simulink model "Kalman_kaskada"  (Simulink 7.8)
settings: Solver=ode45  StartTime=0.0  StopTime=100  RelTol=1e-3
values from neighbouring files (symbols this model uses):
  A = [-1/8 1/8 0 0; 0 -1/10 1/10 0;0 0 -1/1.2 1/1.2; 0 0 0 -1/0.8]    [Parametri.m]
  A1 = [-1/8 1/8 0 0; 0 -1/10 1/10 0;0 0 -1/1.2 1/1.2; 0 0 0 -1/0.8]    [Parametri.m]
  B = [0; 0; 0; 1/0.8]    [Parametri.m]
  B1 = [0; 0; 0; 1/0.8]    [Parametri.m]
  C = [1 0 0 0]    [Parametri.m]
  C1 = [1 0 0 0]    [Parametri.m]
  D = 0    [Parametri.m]
  P1 = 0    [Parametri.m]
  Q = 1*eye(4,4)    [Parametri.m]
  Q1 = 1*eye(4,4)    [Parametri.m]
  R = 1    [Parametri.m]
  R1 = 1    [Parametri.m]
  x0 = [0; 0; 0 ;0]    [Parametri.m]
  x10 = [0; 0; 0 ;0]    [Parametri.m]
undefined symbols (not defined in the file or in its folder): D1
libraries: simulink x4
settings Model: Creator=fo1521  LastModifiedBy=AA
settings OptimizationCC: InitFltsAndDblsToZero=on
settings DebuggingCC: SaveWithParameterizedLinksMsg=none  SolverPrmCheckMsg=none  MultiTaskCondExecSysMsg=none  FcnCallInpInsideContextMsg=Use local settings  StrictBusMsg=None
settings RTWCC: IncludeERTFirstTime=on

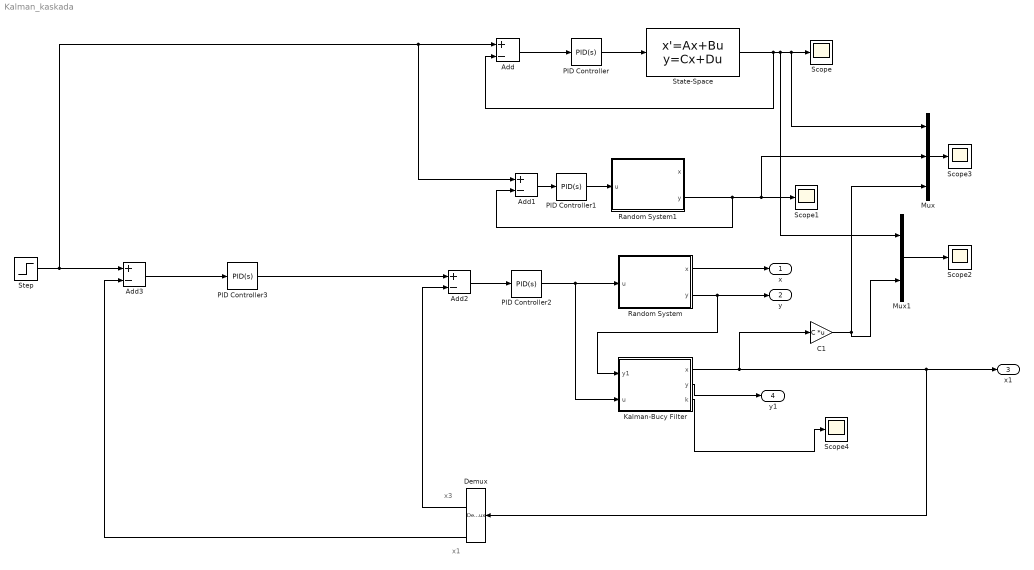
== system Kalman_kaskada ==
  note: x1
  note: x3
  Add{,1..3} (4 alike) : Sum  Inputs=+-
  C1 : Gain  Gain=C  Multiplication=Matrix(K*u)
  Demux : Demux
  Kalman-Bucy Filter : Subsystem  mask{x0=x10, P0=P1, A=A1, B=B1, C=C1, D=D1, Q=Q1, R=R1}
      mask Display:
      | port_label('input',1,'y')
      | port_label('input',2,'u')
      | port_label('output',1,'x')
      | port_label('output',2,'y')
      | disp(sprintf('Kalman-Bucy\n Filter'))
  Mux : Mux  Inputs=3
  Mux1 : Mux  Inputs=2
  PID Controller : simulink/Continuous/PID Controller  Controller=PID  TimeDomain=Continuous-time  SampleTime=1  IntegratorMethod=Forward Euler  FilterMethod=Forward Euler  Form=Parallel  P=2.29954504255598  I=0.157366537101779  D=7.23056950436541  N=1.36221313927971  InitialConditionSource=internal  InitialConditionForIntegrator=0  InitialConditionForFilter=0  ExternalReset=none  LimitOutput=off  UpperSaturationLimit=inf  LowerSaturationLimit=-inf  LinearizeAsGain=off  AntiWindupMode=none  Kb=1  TrackingMode=off  Kt=1  PParamMin=[]  PParamMax=[]  IParamMin=[]  IParamMax=[]  DParamMin=[]  DParamMax=[]  NParamMin=[]  NParamMax=[]  KbParamMin=[]  KbParamMax=[]  KtParamMin=[]  KtParamMax=[]  POutMin=[]  POutMax=[]  IOutMin=[]  IOutMax=[]  DOutMin=[]  DOutMax=[]  NOutMin=[]  NOutMax=[]  KbOutMin=[]  KbOutMax=[]  KtOutMin=[]  KtOutMax=[]  IntegratorOutMin=[]  IntegratorOutMax=[]  FilterOutMin=[]  FilterOutMax=[]  SumOutMin=[]  SumOutMax=[]  SumI1OutMin=[]  SumI1OutMax=[]  SumI2OutMin=[]  SumI2OutMax=[]  SumI3OutMin=[]  SumI3OutMax=[]  SumDOutMin=[]  SumDOutMax=[]  SaturationOutMin=[]  SaturationOutMax=[]  IntegratorContinuousStateAttributes=''  IntegratorStateMustResolveToSignalObject=off  IntegratorRTWStateStorageClass=Auto  FilterContinuousStateAttributes=''  FilterStateMustResolveToSignalObject=off  FilterRTWStateStorageClass=Auto
  PID Controller1 : simulink/Continuous/PID Controller  Controller=PID  TimeDomain=Continuous-time  SampleTime=1  IntegratorMethod=Forward Euler  FilterMethod=Forward Euler  Form=Parallel  P=1  I=1  D=1  N=100  InitialConditionSource=internal  InitialConditionForIntegrator=0  InitialConditionForFilter=0  ExternalReset=none  LimitOutput=off  UpperSaturationLimit=inf  LowerSaturationLimit=-inf  LinearizeAsGain=off  AntiWindupMode=none  Kb=1  TrackingMode=off  Kt=1  PParamMin=[]  PParamMax=[]  IParamMin=[]  IParamMax=[]  DParamMin=[]  DParamMax=[]  NParamMin=[]  NParamMax=[]  KbParamMin=[]  KbParamMax=[]  KtParamMin=[]  KtParamMax=[]  POutMin=[]  POutMax=[]  IOutMin=[]  IOutMax=[]  DOutMin=[]  DOutMax=[]  NOutMin=[]  NOutMax=[]  KbOutMin=[]  KbOutMax=[]  KtOutMin=[]  KtOutMax=[]  IntegratorOutMin=[]  IntegratorOutMax=[]  FilterOutMin=[]  FilterOutMax=[]  SumOutMin=[]  SumOutMax=[]  SumI1OutMin=[]  SumI1OutMax=[]  SumI2OutMin=[]  SumI2OutMax=[]  SumI3OutMin=[]  SumI3OutMax=[]  SumDOutMin=[]  SumDOutMax=[]  SaturationOutMin=[]  SaturationOutMax=[]  IntegratorContinuousStateAttributes=''  IntegratorStateMustResolveToSignalObject=off  IntegratorRTWStateStorageClass=Auto  FilterContinuousStateAttributes=''  FilterStateMustResolveToSignalObject=off  FilterRTWStateStorageClass=Auto
  PID Controller2 : simulink/Continuous/PID Controller  Controller=PID  TimeDomain=Continuous-time  SampleTime=1  IntegratorMethod=Forward Euler  FilterMethod=Forward Euler  Form=Parallel  P=1  I=1  D=1  N=100  InitialConditionSource=internal  InitialConditionForIntegrator=0  InitialConditionForFilter=0  ExternalReset=none  LimitOutput=off  UpperSaturationLimit=inf  LowerSaturationLimit=-inf  LinearizeAsGain=off  AntiWindupMode=none  Kb=1  TrackingMode=off  Kt=1  PParamMin=[]  PParamMax=[]  IParamMin=[]  IParamMax=[]  DParamMin=[]  DParamMax=[]  NParamMin=[]  NParamMax=[]  KbParamMin=[]  KbParamMax=[]  KtParamMin=[]  KtParamMax=[]  POutMin=[]  POutMax=[]  IOutMin=[]  IOutMax=[]  DOutMin=[]  DOutMax=[]  NOutMin=[]  NOutMax=[]  KbOutMin=[]  KbOutMax=[]  KtOutMin=[]  KtOutMax=[]  IntegratorOutMin=[]  IntegratorOutMax=[]  FilterOutMin=[]  FilterOutMax=[]  SumOutMin=[]  SumOutMax=[]  SumI1OutMin=[]  SumI1OutMax=[]  SumI2OutMin=[]  SumI2OutMax=[]  SumI3OutMin=[]  SumI3OutMax=[]  SumDOutMin=[]  SumDOutMax=[]  SaturationOutMin=[]  SaturationOutMax=[]  IntegratorContinuousStateAttributes=''  IntegratorStateMustResolveToSignalObject=off  IntegratorRTWStateStorageClass=Auto  FilterContinuousStateAttributes=''  FilterStateMustResolveToSignalObject=off  FilterRTWStateStorageClass=Auto
  PID Controller3 : simulink/Continuous/PID Controller  Controller=PID  TimeDomain=Continuous-time  SampleTime=1  IntegratorMethod=Forward Euler  FilterMethod=Forward Euler  Form=Parallel  P=1  I=1  D=1  N=100  InitialConditionSource=internal  InitialConditionForIntegrator=0  InitialConditionForFilter=0  ExternalReset=none  LimitOutput=off  UpperSaturationLimit=inf  LowerSaturationLimit=-inf  LinearizeAsGain=off  AntiWindupMode=none  Kb=1  TrackingMode=off  Kt=1  PParamMin=[]  PParamMax=[]  IParamMin=[]  IParamMax=[]  DParamMin=[]  DParamMax=[]  NParamMin=[]  NParamMax=[]  KbParamMin=[]  KbParamMax=[]  KtParamMin=[]  KtParamMax=[]  POutMin=[]  POutMax=[]  IOutMin=[]  IOutMax=[]  DOutMin=[]  DOutMax=[]  NOutMin=[]  NOutMax=[]  KbOutMin=[]  KbOutMax=[]  KtOutMin=[]  KtOutMax=[]  IntegratorOutMin=[]  IntegratorOutMax=[]  FilterOutMin=[]  FilterOutMax=[]  SumOutMin=[]  SumOutMax=[]  SumI1OutMin=[]  SumI1OutMax=[]  SumI2OutMin=[]  SumI2OutMax=[]  SumI3OutMin=[]  SumI3OutMax=[]  SumDOutMin=[]  SumDOutMax=[]  SaturationOutMin=[]  SaturationOutMax=[]  IntegratorContinuousStateAttributes=''  IntegratorStateMustResolveToSignalObject=off  IntegratorRTWStateStorageClass=Auto  FilterContinuousStateAttributes=''  FilterStateMustResolveToSignalObject=off  FilterRTWStateStorageClass=Auto
  Random System : Subsystem  mask{x0=x0, A=A, B=B, C=C, D=D, Q=sqrtm(Q), R=sqrtm(R)}
      mask Display:
      | port_label('input',1,'u')
      | port_label('output',1,'x')
      | port_label('output',2,'y')
      | disp(sprintf('Gassian\n Process'))
  Random System1 : Subsystem  mask{x0=x0, A=A, B=B, C=C, D=D, Q=sqrtm(Q), R=sqrtm(R)}
      mask Display:
      | port_label('input',1,'u')
      | port_label('output',1,'x')
      | port_label('output',2,'y')
      | disp(sprintf('Gassian\n Process'))
  Scope{,1..4} (5 alike) : Scope
      Scope2 settings: YMin=0  YMax=11  SaveName=ScopeData2
      Scope3 settings: SaveName=ScopeData3
      Scope4 settings: SaveName=ScopeData4
  State-Space : StateSpace  A=A  B=B  C=C  D=D  X0=x0
  Step : Step  Time=0  After=10  SampleTime=0
  x : Outport
  y : Outport  Port=2
  x1 : Outport  Port=3
  y1 : Outport  Port=4
  wires:
  PID Controller/1 -> State-Space/1
  State-Space/1 -> Add/2, Scope/1, Mux/1, Mux1/1
  Add/1 -> PID Controller/1
  Random System/1(x) -> x/1
  Random System/2(y) -> Kalman-Bucy Filter/1(y1), y/1
  Kalman-Bucy Filter/1(x) -> C1/1, x1/1, Demux/1
  Kalman-Bucy Filter/2(y) -> y1/1
  Add1/1 -> PID Controller1/1
  PID Controller1/1 -> Random System1/1(u)
  Random System1/2(y) -> Add1/2, Scope1/1, Mux/2
  PID Controller2/1 -> Random System/1(u), Kalman-Bucy Filter/2(u)
  Add2/1 -> PID Controller2/1
  C1/1 -> Mux/3, Mux1/2
  Mux/1 -> Scope3/1
  Kalman-Bucy Filter/3(k) -> Scope4/1
  Demux/2 -> Add2/2
  PID Controller3/1 -> Add2/1
  Step/1 -> Add3/1, Add/1, Add1/1
  Add3/1 -> PID Controller3/1
  Demux/4 -> Add3/2
  Mux1/1 -> Scope2/1

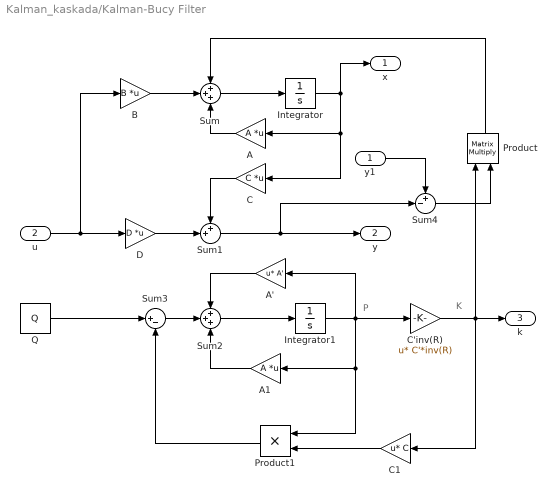
== system Kalman_kaskada/Kalman-Bucy Filter ==
  note: K
  note: P
  y1 : Inport
  u : Inport  Port=2  PortDimensions=size(B,2)
  A : Gain  Gain=A  Multiplication=Matrix(K*u)
  A' : Gain  Gain=A'  Multiplication=Matrix(u*K)
  A1 : Gain  Gain=A  Multiplication=Matrix(K*u)
  B : Gain  Gain=B  Multiplication=Matrix(K*u)
  C : Gain  Gain=C  Multiplication=Matrix(K*u)
  C'inv(R) : Gain  Gain=C'*inv(R)  Multiplication=Matrix(u*K)
  C1 : Gain  Gain=C  Multiplication=Matrix(u*K)
  D : Gain  Gain=D  Multiplication=Matrix(K*u)
  Integrator : Integrator  InitialCondition=x0
  Integrator1 : Integrator  InitialCondition=P0
  Product : Product  Multiplication=Matrix(*)  RndMeth=Zero
  Product1 : Product  RndMeth=Zero
  Q : Constant  Value=Q
  Sum : Sum  Inputs=+++
  Sum1 : Sum  Inputs=++|
  Sum2 : Sum  Inputs=+++
  Sum3 : Sum  Inputs=|+-
  Sum4 : Sum  Inputs=+-|
  x : Outport
  y : Outport  Port=2
  k : Outport  Port=3
  wires:
  Sum1/1 -> y/1, Sum4/2
  D/1 -> Sum1/2
  C/1 -> Sum1/1
  B/1 -> Sum/2
  A/1 -> Sum/3
  Integrator/1 -> x/1, C/1, A/1
  Sum/1 -> Integrator/1
  u/1 -> D/1, B/1
  Sum2/1 -> Integrator1/1
  Integrator1/1 -> A'/1, C'inv(R)/1, A1/1, Product1/1
  A1/1 -> Sum2/3
  A'/1 -> Sum2/1
  Q/1 -> Sum3/1
  Sum3/1 -> Sum2/2
  y1/1 -> Sum4/1
  Product/1 -> Sum/1
  C'inv(R)/1 -> C1/1, Product/1, k/1
  Product1/1 -> Sum3/2
  C1/1 -> Product1/2
  Sum4/1 -> Product/2

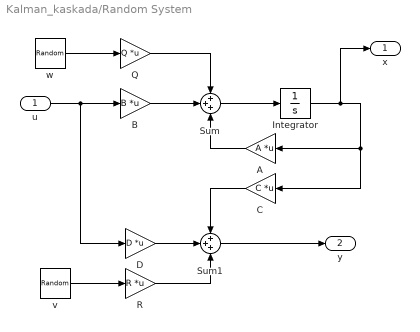
== system Kalman_kaskada/Random System ==
  u : Inport  PortDimensions=size(B,2)
  A : Gain  Gain=A  Multiplication=Matrix(K*u)
  B : Gain  Gain=B  Multiplication=Matrix(K*u)
  C : Gain  Gain=C  Multiplication=Matrix(K*u)
  D : Gain  Gain=D  Multiplication=Matrix(K*u)
  Integrator : Integrator  InitialCondition=x0
  Q : Gain  Gain=Q  Multiplication=Matrix(K*u)
  R : Gain  Gain=R  Multiplication=Matrix(K*u)
  Sum : Sum  Inputs=+++
  Sum1 : Sum  Inputs=+++
  v : RandomNumber  Mean=zeros(size(R,1),1)  Variance=ones(size(R,1),1)  SampleTime=0
  w : RandomNumber  Mean=zeros(numel(x0),1)  Variance=ones(numel(x0),1)  SampleTime=0
  x : Outport
  y : Outport  Port=2
  wires:
  Sum/1 -> Integrator/1
  Integrator/1 -> A/1, C/1, x/1
  A/1 -> Sum/3
  B/1 -> Sum/2
  u/1 -> B/1, D/1
  w/1 -> Q/1
  Q/1 -> Sum/1
  C/1 -> Sum1/1
  D/1 -> Sum1/2
  v/1 -> R/1
  R/1 -> Sum1/3
  Sum1/1 -> y/1

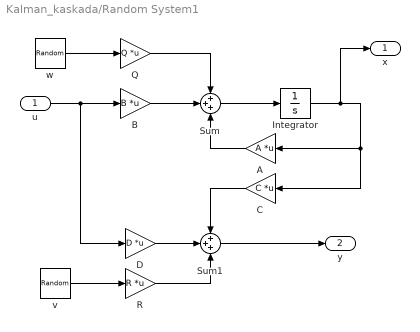
== system Kalman_kaskada/Random System1 ==
  u : Inport  PortDimensions=size(B,2)
  A : Gain  Gain=A  Multiplication=Matrix(K*u)
  B : Gain  Gain=B  Multiplication=Matrix(K*u)
  C : Gain  Gain=C  Multiplication=Matrix(K*u)
  D : Gain  Gain=D  Multiplication=Matrix(K*u)
  Integrator : Integrator  InitialCondition=x0
  Q : Gain  Gain=Q  Multiplication=Matrix(K*u)
  R : Gain  Gain=R  Multiplication=Matrix(K*u)
  Sum : Sum  Inputs=+++
  Sum1 : Sum  Inputs=+++
  v : RandomNumber  Mean=zeros(size(R,1),1)  Variance=ones(size(R,1),1)  SampleTime=0
  w : RandomNumber  Mean=zeros(numel(x0),1)  Variance=ones(numel(x0),1)  SampleTime=0
  x : Outport
  y : Outport  Port=2
  wires:
  Sum1/1 -> y/1
  R/1 -> Sum1/3
  v/1 -> R/1
  D/1 -> Sum1/2
  C/1 -> Sum1/1
  Q/1 -> Sum/1
  w/1 -> Q/1
  u/1 -> D/1, B/1
  B/1 -> Sum/2
  A/1 -> Sum/3
  Integrator/1 -> x/1, C/1, A/1
  Sum/1 -> Integrator/1
